simulink model "simPFuzzy"  (R2023b)
settings: Solver=VariableStepAuto  StartTime=0.0  StopTime=initValues(2)  RelTol=1e-3
values from neighbouring files (symbols this model uses):
  initValues = initialize()    [Comparision.m]    (also in initialize.m = [T, tsim, stepValue, upperLim, lowerLim, K, tau]; programClassic.m; programFuzzy.m)
libraries: fuzblock x1
settings Model: Creator=usuario  LastModifiedBy=usuario
settings DataIOCC: ReturnWorkspaceOutputs=off

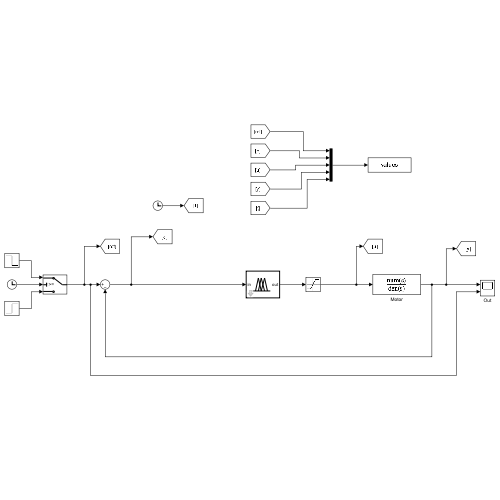
[thumbnail: Simulink's stored preview of the top-level diagram]
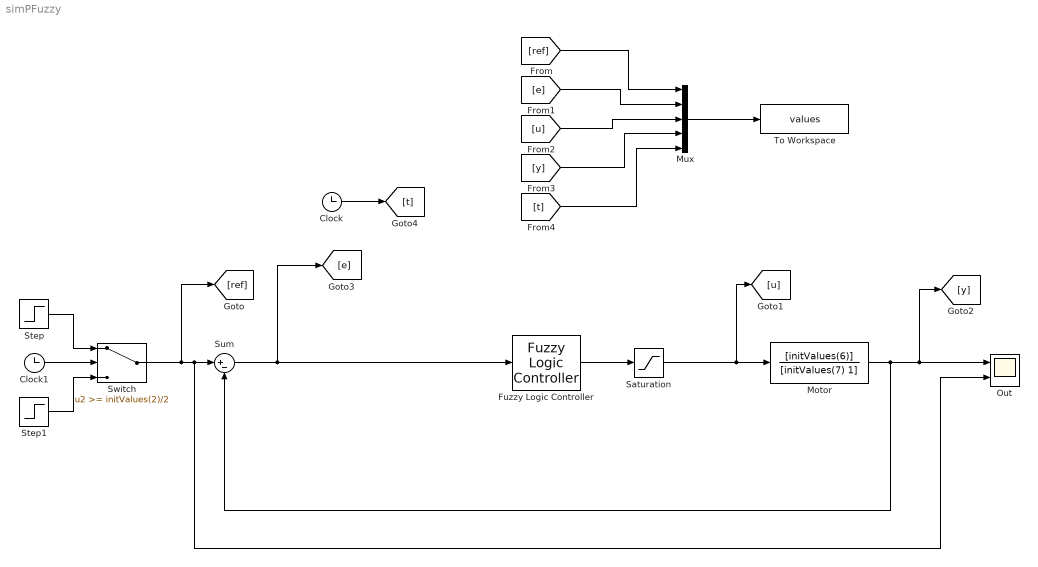
== system simPFuzzy ==
  Clock : Clock
  Clock1 : Clock
  Fuzzy Logic Controller : fuzblock/Fuzzy Logic  Controller  FIS='fuzzyP.fis'  OutputSampleNumber=101  DataType=double  FuzzifiedInputs=off  RuleFiringStrengths=off  RuleOutputs=off  AggregatedOutputs=off  SimulateUsing=Interpreted execution  OutOfRangeInputValueMessage=warning  NoRuleFiredMessage=warning  EmptyOutputFuzzySetMessage=warning
  Motor : TransferFcn  Numerator=[initValues(6)]  Denominator=[initValues(7) 1]
  Mux : Mux  Inputs=5
  Out : Scope  NumInputPorts=2
  Saturation : Saturate  UpperLimit=initValues(4)  LowerLimit=initValues(5)
  Step : Step  After=-initValues(3)  SampleTime=0
  Step1 : Step  After=initValues(3)/2  SampleTime=0
  Sum : Sum  Inputs=|+-
  Switch : Switch  Threshold=initValues(2)/2  SaturateOnIntegerOverflow=off  InputSameDT=off
  To Workspace : ToWorkspace  VariableName=values  SaveFormat=Structure  SampleTime=initValues(1)
  wires:
  Sum/1 -> Fuzzy Logic Controller/1, [e]
  Motor/1 -> Sum/2, [y], Out/1
  Switch/1 -> [ref], Out/2, Sum/1
  [ref] -> Mux/1
  [y] -> Mux/4
  [e] -> Mux/2
  [u] -> Mux/3
  Mux/1 -> To Workspace/1
  Clock/1 -> [t]
  [t] -> Mux/5
  Clock1/1 -> Switch/2
  Step/1 -> Switch/1
  Step1/1 -> Switch/3
  Fuzzy Logic Controller/1 -> Saturation/1
  Saturation/1 -> [u], Motor/1
